simulink model "zeropole_test"  (Simulink 8.4)
settings: Solver=ode45  StartTime=0.0  StopTime=10.0  RelTol=1e-3
libraries: discretizing x1
settings Model: Creator=arnaud  LastModifiedBy=arnaud
settings DataIOCC: SaveFormat=Structure  SignalLoggingSaveFormat=Dataset
settings OptimizationCC: ExpressionDepthLimit=128
settings DebuggingCC: UnderspecifiedInitializationDetection=Simplified  MergeDetectMultiDrivingBlocksExec=error  FcnCallInpInsideContextMsg=EnableAllAsError  StateNameClashWarn=none
settings GRTTargetCC: CombineOutputUpdateFcns=on  GRTInterface=off

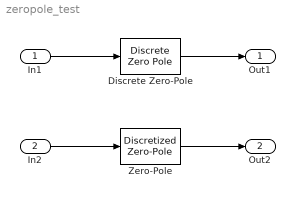
== system zeropole_test ==
  In1 : Inport
  In2 : Inport  Port=2
  Discrete Zero-Pole : DiscreteZeroPole  Poles=[0 0.5]  Gain=1
  Zero-Pole : discretizing/Discretized Zero-Pole  Zeros=[1]  Poles=[0 -1]  Gain=[1]  AbsTol=auto  SampleTime=1.0  method=zoh  Wc=1
  Out1 : Outport
  Out2 : Outport  Port=2
  wires:
  In1/1 -> Discrete Zero-Pole/1
  Discrete Zero-Pole/1 -> Out1/1
  In2/1 -> Zero-Pole/1
  Zero-Pole/1 -> Out2/1
